simulink model "AFDNFSmodelSPA"  (R2017b)
settings: Solver=ode45  StartTime=0.0  StopTime=1400  FixedStep=1e-3  RelTol=1e-8  EnableMultiTasking=on
PostLoadFcn:
  | run('Methods/NFSOnLoad');
InitFcn:
  | run('Methods/AFDSimInit')
StopFcn:
  | run('Methods/NFSOnLoad');
values from neighbouring files (symbols this model uses):
  nfs = TransferFunction('Plot','true')    [Main.m]    (also in NFSDatabase.sldd = SI
                Imperial
                28184.4409185639)
undefined symbols (not defined in the file or in its folder): Continuous, desired, Earth, F, K_lat, K_long, Kobsvlat, Kobsvlong, lat, latsys, Light, long, longsys, MIL, Newton, Raphson, sigbuilder_block, Time, WGS84
libraries: simulink x6, aerolibtransform2 x2, aerolibwind2 x2, ModelsLibrary x1, ctrlSharedLib x1, sharedutil x1
(part 4 of 4)

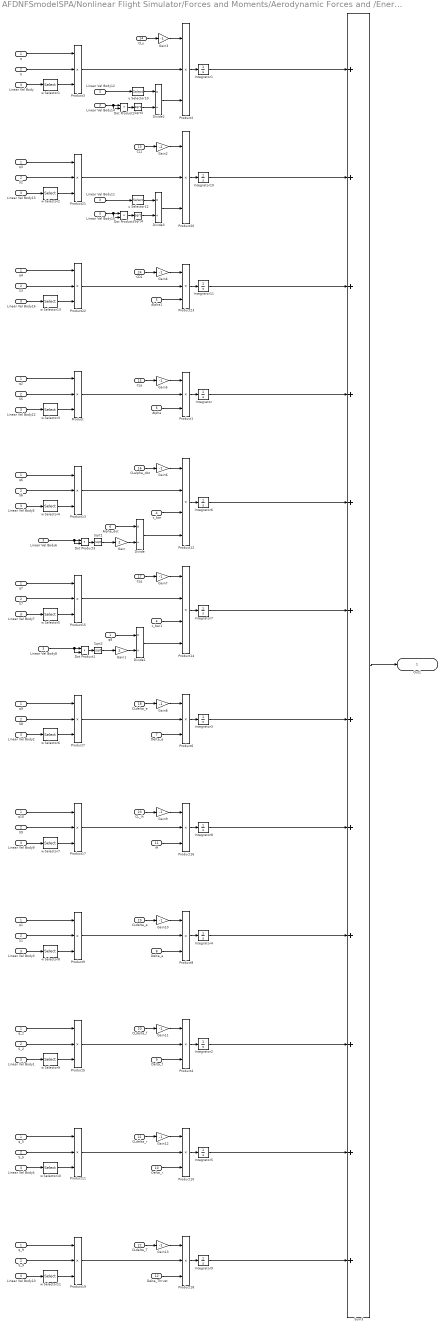
== system AFDNFSmodelSPA/Nonlinear Flight Simulator/Forces and Moments/Aerodynamic Forces and /Energy Analysis1/Longitudinal1/Lift ==
  q : Inport
  S : Inport  Port=2
  Linear Vel Body : Inport  Port=3
  c_bar : Inport  Port=4
  Alpha : Inport  Port=5
  Alpha_dot : Inport  Port=6
  Delta_e : Inport  Port=7
  Delta_a : Inport  Port=8
  Delta_f : Inport  Port=9
  Delta_r : Inport  Port=10
  iH : Inport  Port=11
  Delta_Thrust : Inport  Port=12
  CL1 : Inport  Port=13
  CLu : Inport  Port=14
  CLa : Inport  Port=15
  CLalpha_dot : Inport  Port=16
  CLq : Inport  Port=17
  CLdelta_e : Inport  Port=18
  CLdelta_a : Inport  Port=19
  CLdelta_f : Inport  Port=20
  CLdelta_r : Inport  Port=21
  CLdelta_T : Inport  Port=22
  CL_ih : Inport  Port=23
  CD1 : Inport  Port=24
  Alpha1 : InportShadow  Port=5
  Divide{,1..3} (4 alike) : Product  Inputs=*/
  Dot Product{1..4} (4 alike) : DotProduct  InputSameDT=on  OutDataTypeStr=Inherit: Inherit via internal rule
  Gain : Gain  Gain=2
  Gain1 : Gain  Gain=2
  Gain{3..13} (11 alike) : Gain  Gain=-1
  Gain2 : Gain  Gain=-2
  Integrator{,1..11} (12 alike) : Integrator
  Linear Vel Body{1..16,22} (17 alike) : InportShadow  Port=3
  Product{,1..11,13,15..23} (22 alike) : Product  Inputs=3
  Product12 : Product  Inputs=4
  Product14 : Product  Inputs=4
  S{1..3,5..9} (8 alike) : InportShadow  Port=2
  S_2 : InportShadow  Port=2
  S_5 : InportShadow  Port=2
  S_9 : InportShadow  Port=2
  Sqrt{1..4} (4 alike) : Sqrt  SaturateOnIntegerOverflow=on
  Sum3 : Sum  Inputs=++++++++++++
  c_bar1 : InportShadow  Port=4
  q{1..4,6..10} (9 alike) : InportShadow
  q_2 : InportShadow
  q_5 : InportShadow
  q_9 : InportShadow
  u Selector10 : Selector  InputPortWidth=3  IndexOptions=Index vector (dialog)  Indices=[1]  OutputSizes=1
  u Selector12 : Selector  InputPortWidth=3  IndexOptions=Index vector (dialog)  Indices=[1]  OutputSizes=1
  w Selector{1..11,13} (12 alike) : Selector  InputPortWidth=3  IndexOptions=Index vector (dialog)  Indices=[3]  OutputSizes=1
  Out1 : Outport
  wires:
  Integrator1/1 -> Sum3/1
  CLu/1 -> Gain3/1
  Product3/1 -> Product2/2
  Divide2/1 -> Product2/3
  Product2/1 -> Integrator1/1
  Integrator10/1 -> Sum3/2
  q/1 -> Product3/1
  S/1 -> Product3/2
  Sum3/1 -> Out1/1
  w Selector1/1 -> Product3/3
  Linear Vel Body/1 -> w Selector1/1
  Sqrt3/1 -> Divide2/2
  u Selector10/1 -> Divide2/1
  Dot Product2/1 -> Sqrt3/1
  Linear Vel Body14/1 -> Dot Product2/1, Dot Product2/2
  Linear Vel Body12/1 -> u Selector10/1
  CL1/1 -> Gain2/1
  Product21/1 -> Product20/2
  Divide3/1 -> Product20/3
  Product20/1 -> Integrator10/1
  q3/1 -> Product21/1
  S2/1 -> Product21/2
  w Selector2/1 -> Product21/3
  Linear Vel Body13/1 -> w Selector2/1
  Sqrt4/1 -> Divide3/2
  u Selector12/1 -> Divide3/1
  Dot Product4/1 -> Sqrt4/1
  Linear Vel Body15/1 -> Dot Product4/2, Dot Product4/1
  Linear Vel Body11/1 -> u Selector12/1
  Gain2/1 -> Product20/1
  Integrator6/1 -> Sum3/5
  Integrator3/1 -> Sum3/7
  Integrator4/1 -> Sum3/9
  Integrator2/1 -> Sum3/10
  Integrator5/1 -> Sum3/11
  CLdelta_T/1 -> Gain13/1
  Product19/1 -> Product18/2
  Delta_Thrust/1 -> Product18/3
  Product18/1 -> Integrator9/1
  q_9/1 -> Product19/1
  S_9/1 -> Product19/2
  w Selector11/1 -> Product19/3
  Linear Vel Body10/1 -> w Selector11/1
  Integrator9/1 -> Sum3/12
  CLdelta_r/1 -> Gain12/1
  Product11/1 -> Product10/2
  Delta_r/1 -> Product10/3
  Product10/1 -> Integrator5/1
  q_5/1 -> Product11/1
  S_5/1 -> Product11/2
  w Selector10/1 -> Product11/3
  Linear Vel Body4/1 -> w Selector10/1
  CLdelta_f/1 -> Gain11/1
  Product5/1 -> Product4/2
  Delta_f/1 -> Product4/3
  Product4/1 -> Integrator2/1
  q_2/1 -> Product5/1
  S_2/1 -> Product5/2
  w Selector9/1 -> Product5/3
  Linear Vel Body1/1 -> w Selector9/1
  Alpha/1 -> Product1/3
  CLa/1 -> Gain5/1
  Product/1 -> Product1/2
  Product1/1 -> Integrator/1
  q2/1 -> Product/1
  S5/1 -> Product/2
  Linear Vel Body22/1 -> w Selector3/1
  w Selector3/1 -> Product/3
  CLdelta_e/1 -> Gain8/1
  Product7/1 -> Product6/2
  Delta_e/1 -> Product6/3
  Product6/1 -> Integrator3/1
  q9/1 -> Product7/1
  S8/1 -> Product7/2
  w Selector6/1 -> Product7/3
  Linear Vel Body2/1 -> w Selector6/1
  CLdelta_a/1 -> Gain10/1
  Product9/1 -> Product8/2
  Delta_a/1 -> Product8/3
  Product8/1 -> Integrator4/1
  q1/1 -> Product9/1
  S1/1 -> Product9/2
  w Selector8/1 -> Product9/3
  Linear Vel Body3/1 -> w Selector8/1
  CLalpha_dot/1 -> Gain6/1
  Product13/1 -> Product12/2
  c_bar/1 -> Product12/3
  Product12/1 -> Integrator6/1
  q6/1 -> Product13/1
  S6/1 -> Product13/2
  w Selector4/1 -> Product13/3
  Linear Vel Body5/1 -> w Selector4/1
  Gain/1 -> Divide/2
  Alpha_dot/1 -> Divide/1
  Divide/1 -> Product12/4
  Dot Product3/1 -> Sqrt1/1
  Linear Vel Body6/1 -> Dot Product3/1, Dot Product3/2
  Sqrt1/1 -> Gain/1
  CLq/1 -> Gain7/1
  Product15/1 -> Product14/2
  c_bar1/1 -> Product14/3
  Product14/1 -> Integrator7/1
  q7/1 -> Product15/1
  S7/1 -> Product15/2
  w Selector5/1 -> Product15/3
  Linear Vel Body7/1 -> w Selector5/1
  Gain1/1 -> Divide1/2
  q8/1 -> Divide1/1
  Divide1/1 -> Product14/4
  Dot Product1/1 -> Sqrt2/1
  Linear Vel Body8/1 -> Dot Product1/2, Dot Product1/1
  Sqrt2/1 -> Gain1/1
  CL_ih/1 -> Gain9/1
  Product17/1 -> Product16/2
  iH/1 -> Product16/3
  Product16/1 -> Integrator8/1
  q10/1 -> Product17/1
  S9/1 -> Product17/2
  w Selector7/1 -> Product17/3
  Linear Vel Body9/1 -> w Selector7/1
  Integrator8/1 -> Sum3/8
  Integrator/1 -> Sum3/4
  Integrator7/1 -> Sum3/6
  Alpha1/1 -> Product23/3
  CD1/1 -> Gain4/1
  Product22/1 -> Product23/2
  Product23/1 -> Integrator11/1
  q4/1 -> Product22/1
  S3/1 -> Product22/2
  Linear Vel Body16/1 -> w Selector13/1
  w Selector13/1 -> Product22/3
  Integrator11/1 -> Sum3/3
  Gain3/1 -> Product2/1
  Gain4/1 -> Product23/1
  Gain5/1 -> Product1/1
  Gain6/1 -> Product12/1
  Gain7/1 -> Product14/1
  Gain8/1 -> Product6/1
  Gain9/1 -> Product16/1
  Gain10/1 -> Product8/1
  Gain11/1 -> Product4/1
  Gain12/1 -> Product10/1
  Gain13/1 -> Product18/1

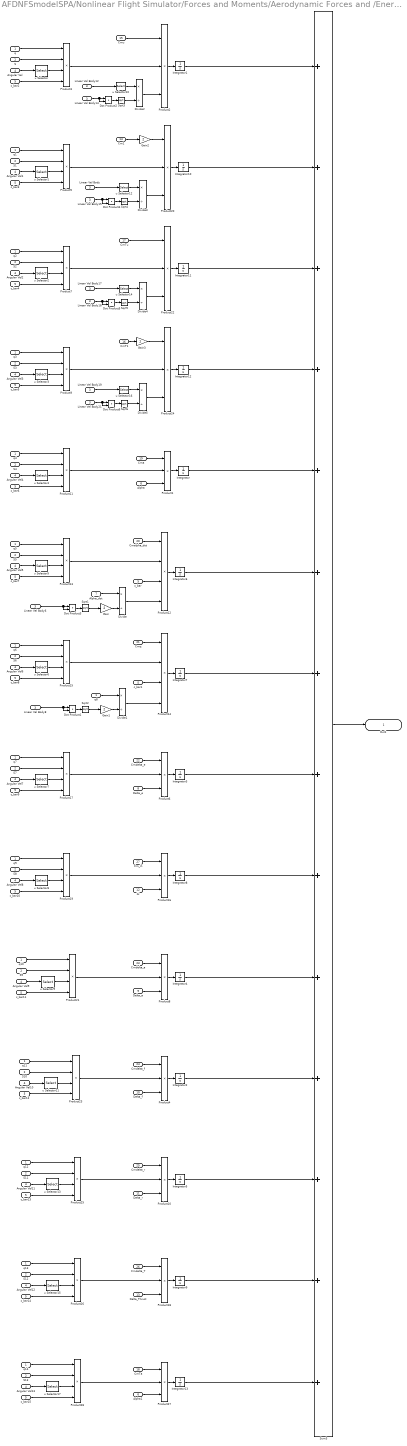
== system AFDNFSmodelSPA/Nonlinear Flight Simulator/Forces and Moments/Aerodynamic Forces and /Energy Analysis1/Longitudinal1/Pitch ==
  q : Inport
  S : Inport  Port=2
  Linear Vel Body : Inport  Port=3
  Angular Vel : Inport  Port=4
  c_bar : Inport  Port=5
  Alpha : Inport  Port=6
  Alpha_dot : Inport  Port=7
  Delta_e : Inport  Port=8
  Delta_a : Inport  Port=9
  Delta_f : Inport  Port=10
  Delta_r : Inport  Port=11
  iH : Inport  Port=12
  Delta_Thrust : Inport  Port=13
  Cm1 : Inport  Port=14
  Cmu : Inport  Port=15
  CmT1 : Inport  Port=16
  CmTu : Inport  Port=17
  CmTa : Inport  Port=18
  Cma : Inport  Port=19
  Cmalpha_dot : Inport  Port=20
  Cmq : Inport  Port=21
  Cmdelta_e : Inport  Port=22
  Cmdelta_a : Inport  Port=23
  Cmdelta_f : Inport  Port=24
  Cmdelta_r : Inport  Port=25
  Cmdelta_T : Inport  Port=26
  Cm_ih : Inport  Port=27
  Alpha1 : InportShadow  Port=6
  Angular Vel{1..13} (13 alike) : InportShadow  Port=4
  Divide{,1..5} (6 alike) : Product  Inputs=*/
  Dot Product{1..6} (6 alike) : DotProduct  InputSameDT=on  OutDataTypeStr=Inherit: Inherit via internal rule
  Gain{,1..3} (4 alike) : Gain  Gain=2
  Integrator{,1..13} (14 alike) : Integrator
  Linear Vel Body{6,8,12,14..15,17..19,21} (9 alike) : InportShadow  Port=3
  Product{1..2,4,6,8,10,16,18,20,22,24,27} (12 alike) : Product  Inputs=3
  Product{3,5,7,9,11..15,17,19,21,23,25..26,28} (16 alike) : Product  Inputs=4
  S{1..13} (13 alike) : InportShadow  Port=2
  Sqrt{1..6} (6 alike) : Sqrt  SaturateOnIntegerOverflow=on
  Sum3 : Sum  Inputs=++++++++++++++
  c_bar{1..15} (15 alike) : InportShadow  Port=5
  q{1..14} (14 alike) : InportShadow
  u Selector{,1..9,11,13,15,17} (14 alike) : Selector  InputPortWidth=3  IndexOptions=Index vector (dialog)  Indices=[2]  OutputSizes=1
  u Selector{10,12,14,16} (4 alike) : Selector  InputPortWidth=3  IndexOptions=Index vector (dialog)  Indices=[1]  OutputSizes=1
  Out1 : Outport
  wires:
  Integrator7/1 -> Sum3/7
  Integrator12/1 -> Sum3/4
  Gain3/1 -> Product24/1
  Linear Vel Body19/1 -> u Selector16/1
  Linear Vel Body21/1 -> Dot Product6/1, Dot Product6/2
  Dot Product6/1 -> Sqrt6/1
  u Selector16/1 -> Divide5/1
  Sqrt6/1 -> Divide5/2
  Product24/1 -> Integrator12/1
  Divide5/1 -> Product24/3
  Product9/1 -> Product24/2
  CmT1/1 -> Gain3/1
  Integrator11/1 -> Sum3/3
  Linear Vel Body17/1 -> u Selector14/1
  Linear Vel Body18/1 -> Dot Product5/2, Dot Product5/1
  Dot Product5/1 -> Sqrt5/1
  u Selector14/1 -> Divide4/1
  Sqrt5/1 -> Divide4/2
  Product22/1 -> Integrator11/1
  Divide4/1 -> Product22/3
  Product7/1 -> Product22/2
  CmTu/1 -> Product22/1
  Gain2/1 -> Product20/1
  Linear Vel Body/1 -> u Selector12/1
  Linear Vel Body15/1 -> Dot Product4/1, Dot Product4/2
  Dot Product4/1 -> Sqrt4/1
  u Selector12/1 -> Divide3/1
  Sqrt4/1 -> Divide3/2
  Product20/1 -> Integrator10/1
  Divide3/1 -> Product20/3
  Product5/1 -> Product20/2
  Cm1/1 -> Gain2/1
  Integrator/1 -> Sum3/5
  Integrator8/1 -> Sum3/9
  Product16/1 -> Integrator8/1
  iH/1 -> Product16/3
  Product19/1 -> Product16/2
  Cm_ih/1 -> Product16/1
  Sqrt2/1 -> Gain1/1
  Linear Vel Body8/1 -> Dot Product1/1, Dot Product1/2
  Dot Product1/1 -> Sqrt2/1
  Divide1/1 -> Product14/4
  q8/1 -> Divide1/1
  Gain1/1 -> Divide1/2
  Product14/1 -> Integrator7/1
  c_bar1/1 -> Product14/3
  Product15/1 -> Product14/2
  Cmq/1 -> Product14/1
  Sqrt1/1 -> Gain/1
  Linear Vel Body6/1 -> Dot Product3/2, Dot Product3/1
  Dot Product3/1 -> Sqrt1/1
  Divide/1 -> Product12/4
  Alpha_dot/1 -> Divide/1
  Gain/1 -> Divide/2
  Product12/1 -> Integrator6/1
  c_bar/1 -> Product12/3
  Product13/1 -> Product12/2
  Cmalpha_dot/1 -> Product12/1
  Product8/1 -> Integrator4/1
  Delta_a/1 -> Product8/3
  Product21/1 -> Product8/2
  Cmdelta_a/1 -> Product8/1
  Product6/1 -> Integrator3/1
  Delta_e/1 -> Product6/3
  Product17/1 -> Product6/2
  Cmdelta_e/1 -> Product6/1
  Product1/1 -> Integrator/1
  Product11/1 -> Product1/2
  Cma/1 -> Product1/1
  Alpha/1 -> Product1/3
  Product4/1 -> Integrator2/1
  Delta_f/1 -> Product4/3
  Product23/1 -> Product4/2
  Cmdelta_f/1 -> Product4/1
  Product10/1 -> Integrator5/1
  Delta_r/1 -> Product10/3
  Product25/1 -> Product10/2
  Cmdelta_r/1 -> Product10/1
  Integrator9/1 -> Sum3/13
  Product18/1 -> Integrator9/1
  Delta_Thrust/1 -> Product18/3
  Product26/1 -> Product18/2
  Cmdelta_T/1 -> Product18/1
  Integrator5/1 -> Sum3/12
  Integrator2/1 -> Sum3/11
  Integrator4/1 -> Sum3/10
  Integrator3/1 -> Sum3/8
  Integrator6/1 -> Sum3/6
  Linear Vel Body12/1 -> u Selector10/1
  Linear Vel Body14/1 -> Dot Product2/2, Dot Product2/1
  Dot Product2/1 -> Sqrt3/1
  u Selector10/1 -> Divide2/1
  Sqrt3/1 -> Divide2/2
  Angular Vel/1 -> u Selector/1
  u Selector/1 -> Product3/3
  Sum3/1 -> Out1/1
  S/1 -> Product3/2
  q/1 -> Product3/1
  Integrator10/1 -> Sum3/2
  Product2/1 -> Integrator1/1
  Divide2/1 -> Product2/3
  Product3/1 -> Product2/2
  Integrator1/1 -> Sum3/1
  CmTa/1 -> Product27/1
  Product28/1 -> Product27/2
  Product27/1 -> Integrator13/1
  Alpha1/1 -> Product27/3
  Integrator13/1 -> Sum3/14
  c_bar2/1 -> Product3/4
  Angular Vel1/1 -> u Selector1/1
  u Selector1/1 -> Product5/3
  S1/1 -> Product5/2
  q1/1 -> Product5/1
  c_bar3/1 -> Product5/4
  Angular Vel2/1 -> u Selector2/1
  u Selector2/1 -> Product7/3
  S2/1 -> Product7/2
  q2/1 -> Product7/1
  c_bar4/1 -> Product7/4
  Angular Vel3/1 -> u Selector3/1
  u Selector3/1 -> Product9/3
  S3/1 -> Product9/2
  q3/1 -> Product9/1
  c_bar5/1 -> Product9/4
  Angular Vel4/1 -> u Selector4/1
  u Selector4/1 -> Product11/3
  S4/1 -> Product11/2
  q4/1 -> Product11/1
  c_bar6/1 -> Product11/4
  Angular Vel5/1 -> u Selector5/1
  u Selector5/1 -> Product13/3
  S5/1 -> Product13/2
  q5/1 -> Product13/1
  c_bar7/1 -> Product13/4
  Angular Vel6/1 -> u Selector6/1
  u Selector6/1 -> Product15/3
  S6/1 -> Product15/2
  q6/1 -> Product15/1
  c_bar8/1 -> Product15/4
  Angular Vel7/1 -> u Selector7/1
  u Selector7/1 -> Product17/3
  S7/1 -> Product17/2
  q7/1 -> Product17/1
  c_bar9/1 -> Product17/4
  Angular Vel8/1 -> u Selector8/1
  u Selector8/1 -> Product19/3
  S8/1 -> Product19/2
  q9/1 -> Product19/1
  c_bar10/1 -> Product19/4
  Angular Vel9/1 -> u Selector9/1
  u Selector9/1 -> Product21/3
  S9/1 -> Product21/2
  q10/1 -> Product21/1
  c_bar11/1 -> Product21/4
  Angular Vel10/1 -> u Selector11/1
  u Selector11/1 -> Product23/3
  S10/1 -> Product23/2
  q11/1 -> Product23/1
  c_bar12/1 -> Product23/4
  Angular Vel11/1 -> u Selector13/1
  u Selector13/1 -> Product25/3
  S11/1 -> Product25/2
  q12/1 -> Product25/1
  c_bar13/1 -> Product25/4
  Angular Vel12/1 -> u Selector15/1
  u Selector15/1 -> Product26/3
  S12/1 -> Product26/2
  q13/1 -> Product26/1
  c_bar14/1 -> Product26/4
  Angular Vel13/1 -> u Selector17/1
  u Selector17/1 -> Product28/3
  S13/1 -> Product28/2
  q14/1 -> Product28/1
  c_bar15/1 -> Product28/4
  Cmu/1 -> Product2/1

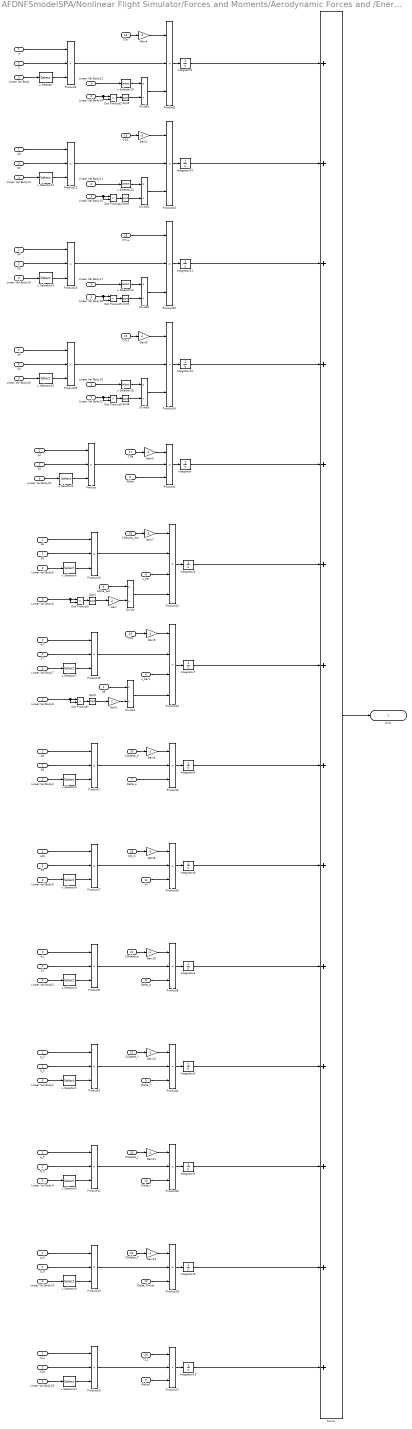
== system AFDNFSmodelSPA/Nonlinear Flight Simulator/Forces and Moments/Aerodynamic Forces and /Energy Analysis1/Longitudinal1/drag ==
  q : Inport
  S : Inport  Port=2
  Linear Vel Body : Inport  Port=3
  c_bar : Inport  Port=4
  Alpha : Inport  Port=5
  Alpha_dot : Inport  Port=6
  Delta_e : Inport  Port=7
  Delta_a : Inport  Port=8
  Delta_f : Inport  Port=9
  Delta_r : Inport  Port=10
  iH : Inport  Port=11
  Delta_Thrust : Inport  Port=12
  CD1 : Inport  Port=13
  CDu : Inport  Port=14
  CTx1 : Inport  Port=15
  CTxu : Inport  Port=16
  CDa : Inport  Port=17
  CDalpha_dot : Inport  Port=18
  CDq : Inport  Port=19
  CDdelta_e : Inport  Port=20
  CDdelta_a : Inport  Port=21
  CDdelta_f : Inport  Port=22
  CDdelta_r : Inport  Port=23
  CDdelta_T : Inport  Port=24
  CD_ih : Inport  Port=25
  CL1 : Inport  Port=26
  Alpha1 : InportShadow  Port=5
  Divide{,1..5} (6 alike) : Product  Inputs=*/
  Dot Product{1..6} (6 alike) : DotProduct  InputSameDT=on  OutDataTypeStr=Inherit: Inherit via internal rule
  Gain : Gain  Gain=2
  Gain1 : Gain  Gain=2
  Gain{4..13} (10 alike) : Gain  Gain=-1
  Gain2 : Gain  Gain=-2
  Gain3 : Gain  Gain=2
  Integrator{,1..13} (14 alike) : Integrator
  Linear Vel Body{1..23} (23 alike) : InportShadow  Port=3
  Product{,1..11,13,15..27} (26 alike) : Product  Inputs=3
  Product12 : Product  Inputs=4
  Product14 : Product  Inputs=4
  S{1..10} (10 alike) : InportShadow  Port=2
  S_2 : InportShadow  Port=2
  S_5 : InportShadow  Port=2
  S_9 : InportShadow  Port=2
  Sqrt{1..6} (6 alike) : Sqrt  SaturateOnIntegerOverflow=on
  Sum3 : Sum  Inputs=++++++++++++++
  c_bar1 : InportShadow  Port=4
  q{1..11} (11 alike) : InportShadow
  q_2 : InportShadow
  q_5 : InportShadow
  q_9 : InportShadow
  u Selector{,1..17} (18 alike) : Selector  InputPortWidth=3  IndexOptions=Index vector (dialog)  Indices=[1]  OutputSizes=1
  Out1 : Outport
  wires:
  Integrator1/1 -> Sum3/1
  CDu/1 -> Gain4/1
  Product3/1 -> Product2/2
  Divide2/1 -> Product2/3
  Product2/1 -> Integrator1/1
  Integrator10/1 -> Sum3/2
  q/1 -> Product3/1
  S/1 -> Product3/2
  Sum3/1 -> Out1/1
  u Selector/1 -> Product3/3
  Linear Vel Body/1 -> u Selector/1
  Sqrt3/1 -> Divide2/2
  u Selector10/1 -> Divide2/1
  Dot Product2/1 -> Sqrt3/1
  Linear Vel Body14/1 -> Dot Product2/1, Dot Product2/2
  Linear Vel Body12/1 -> u Selector10/1
  Integrator6/1 -> Sum3/6
  Integrator3/1 -> Sum3/8
  Integrator4/1 -> Sum3/10
  Integrator2/1 -> Sum3/11
  Integrator5/1 -> Sum3/12
  CDdelta_T/1 -> Gain13/1
  Product19/1 -> Product18/2
  Delta_Thrust/1 -> Product18/3
  Product18/1 -> Integrator9/1
  q_9/1 -> Product19/1
  S_9/1 -> Product19/2
  u Selector9/1 -> Product19/3
  Linear Vel Body10/1 -> u Selector9/1
  Integrator9/1 -> Sum3/13
  CDdelta_r/1 -> Gain11/1
  Product11/1 -> Product10/2
  Delta_r/1 -> Product10/3
  Product10/1 -> Integrator5/1
  q_5/1 -> Product11/1
  S_5/1 -> Product11/2
  u Selector5/1 -> Product11/3
  Linear Vel Body4/1 -> u Selector5/1
  CDdelta_f/1 -> Gain12/1
  Product5/1 -> Product4/2
  Delta_f/1 -> Product4/3
  Product4/1 -> Integrator2/1
  q_2/1 -> Product5/1
  S_2/1 -> Product5/2
  u Selector1/1 -> Product5/3
  Linear Vel Body1/1 -> u Selector1/1
  Alpha/1 -> Product1/3
  CDa/1 -> Gain5/1
  Product/1 -> Product1/2
  Product1/1 -> Integrator/1
  q2/1 -> Product/1
  S5/1 -> Product/2
  Linear Vel Body22/1 -> u Selector2/1
  u Selector2/1 -> Product/3
  CDdelta_e/1 -> Gain6/1
  Product7/1 -> Product6/2
  Delta_e/1 -> Product6/3
  Product6/1 -> Integrator3/1
  q9/1 -> Product7/1
  S8/1 -> Product7/2
  u Selector3/1 -> Product7/3
  Linear Vel Body2/1 -> u Selector3/1
  CDdelta_a/1 -> Gain10/1
  Product9/1 -> Product8/2
  Delta_a/1 -> Product8/3
  Product8/1 -> Integrator4/1
  q1/1 -> Product9/1
  S1/1 -> Product9/2
  u Selector4/1 -> Product9/3
  Linear Vel Body3/1 -> u Selector4/1
  CDalpha_dot/1 -> Gain7/1
  Product13/1 -> Product12/2
  c_bar/1 -> Product12/3
  Product12/1 -> Integrator6/1
  q6/1 -> Product13/1
  S6/1 -> Product13/2
  u Selector6/1 -> Product13/3
  Linear Vel Body5/1 -> u Selector6/1
  Gain/1 -> Divide/2
  Alpha_dot/1 -> Divide/1
  Divide/1 -> Product12/4
  Dot Product3/1 -> Sqrt1/1
  Linear Vel Body6/1 -> Dot Product3/1, Dot Product3/2
  Sqrt1/1 -> Gain/1
  CDq/1 -> Gain9/1
  Product15/1 -> Product14/2
  c_bar1/1 -> Product14/3
  Product14/1 -> Integrator7/1
  q7/1 -> Product15/1
  S7/1 -> Product15/2
  u Selector7/1 -> Product15/3
  Linear Vel Body7/1 -> u Selector7/1
  Gain1/1 -> Divide1/2
  q8/1 -> Divide1/1
  Divide1/1 -> Product14/4
  Dot Product1/1 -> Sqrt2/1
  Linear Vel Body8/1 -> Dot Product1/2, Dot Product1/1
  Sqrt2/1 -> Gain1/1
  CD_ih/1 -> Gain8/1
  Product17/1 -> Product16/2
  iH/1 -> Product16/3
  Product16/1 -> Integrator8/1
  q10/1 -> Product17/1
  S9/1 -> Product17/2
  u Selector8/1 -> Product17/3
  Linear Vel Body9/1 -> u Selector8/1
  Integrator8/1 -> Sum3/9
  Integrator/1 -> Sum3/5
  CD1/1 -> Gain2/1
  Product21/1 -> Product20/2
  Divide3/1 -> Product20/3
  Product20/1 -> Integrator10/1
  q3/1 -> Product21/1
  S2/1 -> Product21/2
  u Selector11/1 -> Product21/3
  Linear Vel Body13/1 -> u Selector11/1
  Sqrt4/1 -> Divide3/2
  u Selector12/1 -> Divide3/1
  Dot Product4/1 -> Sqrt4/1
  Linear Vel Body15/1 -> Dot Product4/2, Dot Product4/1
  Linear Vel Body11/1 -> u Selector12/1
  Gain2/1 -> Product20/1
  CTxu/1 -> Product22/1
  Product23/1 -> Product22/2
  Divide4/1 -> Product22/3
  Product22/1 -> Integrator11/1
  q4/1 -> Product23/1
  S3/1 -> Product23/2
  u Selector13/1 -> Product23/3
  Linear Vel Body16/1 -> u Selector13/1
  Sqrt5/1 -> Divide4/2
  u Selector14/1 -> Divide4/1
  Dot Product5/1 -> Sqrt5/1
  Linear Vel Body18/1 -> Dot Product5/1, Dot Product5/2
  Linear Vel Body17/1 -> u Selector14/1
  Integrator11/1 -> Sum3/3
  CTx1/1 -> Gain3/1
  Product25/1 -> Product24/2
  Divide5/1 -> Product24/3
  Product24/1 -> Integrator12/1
  q5/1 -> Product25/1
  S4/1 -> Product25/2
  u Selector15/1 -> Product25/3
  Linear Vel Body20/1 -> u Selector15/1
  Sqrt6/1 -> Divide5/2
  u Selector16/1 -> Divide5/1
  Dot Product6/1 -> Sqrt6/1
  Linear Vel Body21/1 -> Dot Product6/2, Dot Product6/1
  Linear Vel Body19/1 -> u Selector16/1
  Gain3/1 -> Product24/1
  Integrator12/1 -> Sum3/4
  Integrator7/1 -> Sum3/7
  Alpha1/1 -> Product27/3
  CL1/1 -> Product27/1
  Product26/1 -> Product27/2
  Product27/1 -> Integrator13/1
  q11/1 -> Product26/1
  S10/1 -> Product26/2
  Linear Vel Body23/1 -> u Selector17/1
  u Selector17/1 -> Product26/3
  Integrator13/1 -> Sum3/14
  Gain4/1 -> Product2/1
  Gain5/1 -> Product1/1
  Gain6/1 -> Product6/1
  Gain7/1 -> Product12/1
  Gain9/1 -> Product14/1
  Gain8/1 -> Product16/1
  Gain10/1 -> Product8/1
  Gain12/1 -> Product4/1
  Gain11/1 -> Product10/1
  Gain13/1 -> Product18/1

== system AFDNFSmodelSPA/Nonlinear Flight Simulator/Forces and Moments/Aerodynamic Forces and /Forces/Aerodynamic Forces/Wind2Body TM ==
  Alpha : Inport  PortDimensions=1
  Beta : Inport  Port=2  PortDimensions=1
  ChSign : Gain  Gain=-1  SaturateOnIntegerOverflow=on  OutDataTypeStr=Inherit: Same as input  ParamDataTypeStr=Inherit: Same as input
  ChSign1 : Gain  Gain=-1  SaturateOnIntegerOverflow=on  OutDataTypeStr=Inherit: Same as input  ParamDataTypeStr=Inherit: Same as input
  ChSign2 : Gain  Gain=-1  SaturateOnIntegerOverflow=on  OutDataTypeStr=Inherit: Same as input  ParamDataTypeStr=Inherit: Same as input
  Product{,1..3} (4 alike) : Product  SaturateOnIntegerOverflow=on  InputSameDT=on  OutDataTypeStr=Inherit: Same as first input
  S Matrix : Concatenate  NumInputs=3  Mode=Multidimensional array  ConcatenateDimension=2
  S Col1 : Concatenate  NumInputs=3  Mode=Multidimensional array
  S Col2 : Concatenate  NumInputs=3  Mode=Multidimensional array
  S Col3 : Concatenate  NumInputs=3  Mode=Multidimensional array
  Trigonometric Function : Trigonometry
  Trigonometric Function1 : Trigonometry  Operator=cos
  Trigonometric Function2 : Trigonometry
  Trigonometric Function3 : Trigonometry  Operator=cos
  Zero : Constant  Value=0
  T_BW : Outport  PortDimensions=[3,3]
  wires:
  S Matrix/1 -> T_BW/1
  S Col3/1 -> S Matrix/3
  S Col2/1 -> S Matrix/2
  S Col1/1 -> S Matrix/1
  ChSign2/1 -> S Col3/2
  Product2/1 -> S Col3/1
  Product3/1 -> ChSign2/1
  Zero/1 -> S Col2/3
  ChSign1/1 -> S Col1/3
  ChSign/1 -> S Col1/2
  Product/1 -> S Col1/1
  Product1/1 -> ChSign/1
  Trigonometric Function3/1 -> Product2/2, S Col2/2, Product/2
  Trigonometric Function2/1 -> Product3/2, S Col2/1, Product1/2
  Trigonometric Function1/1 -> Product/1, S Col3/3, Product1/1
  Trigonometric Function/1 -> Product3/1, Product2/1, ChSign1/1
  Beta/1 -> Trigonometric Function2/1, Trigonometric Function3/1
  Alpha/1 -> Trigonometric Function1/1, Trigonometric Function/1

== system AFDNFSmodelSPA/Nonlinear Flight Simulator/Forces and Moments/Aerodynamic Forces and /Forces/Force Coefficients Calculator/Drag Coefficient ==
  CL : Inport  PortDimensions=1
  alpha : Inport  Port=2  PortDimensions=1
  DeltaElevator : Inport  Port=3  PortDimensions=1
  DeltaFlap : Inport  Port=4  PortDimensions=1
  DeltaAileron : Inport  Port=5  PortDimensions=1
  DeltaRudder : Inport  Port=6  PortDimensions=1
  Mach : Inport  Port=7  PortDimensions=1
  Abs{,1..4} (5 alike) : Abs  SaturateOnIntegerOverflow=on
  CD0 : Constant  Value=cD0
  CL^2 : Math  Operator=square  SaturateOnIntegerOverflow=on
  Induced Drag : Gain  Gain=nfs.aero.k  SaturateOnIntegerOverflow=on  OutDataTypeStr=Inherit: Same as input  ParamDataTypeStr=Inherit: Same as input
  Sum2 : Sum  Inputs=++++++++  SaturateOnIntegerOverflow=on  InputSameDT=on  OutDataTypeStr=Inherit: Same as first input
  cDM : Gain  Gain=nfs.aero.cDM  SaturateOnIntegerOverflow=on  OutDataTypeStr=Inherit: Same as input  ParamDataTypeStr=Inherit: Same as input
  cDalpha : Gain  Gain=nfs.aero.cDalpha  SaturateOnIntegerOverflow=on  OutDataTypeStr=Inherit: Same as input  ParamDataTypeStr=Inherit: Same as input
  cDdelta_a : Gain  Gain=nfs.aero.cDdelta_a  SaturateOnIntegerOverflow=on  OutDataTypeStr=Inherit: Same as input  ParamDataTypeStr=Inherit: Same as input
  cDdelta_e : Gain  Gain=nfs.aero.cDdelta_e  SaturateOnIntegerOverflow=on  OutDataTypeStr=Inherit: Same as input  ParamDataTypeStr=Inherit: Same as input
  cDdelta_f : Gain  Gain=nfs.aero.cDdelta_f  SaturateOnIntegerOverflow=on  OutDataTypeStr=Inherit: Same as input  ParamDataTypeStr=Inherit: Same as input
  cDdelta_r : Gain  Gain=nfs.aero.cDdelta_r  SaturateOnIntegerOverflow=on  OutDataTypeStr=Inherit: Same as input  ParamDataTypeStr=Inherit: Same as input
  CD : Outport  PortDimensions=1
  wires:
  Sum2/1 -> CD/1
  DeltaRudder/1 -> cDdelta_r/1
  DeltaAileron/1 -> cDdelta_a/1
  DeltaElevator/1 -> cDdelta_e/1
  DeltaFlap/1 -> cDdelta_f/1
  Mach/1 -> cDM/1
  CL/1 -> CL^2/1
  cDdelta_r/1 -> Abs3/1
  cDdelta_a/1 -> Abs2/1
  cDdelta_e/1 -> Abs1/1
  cDdelta_f/1 -> Abs/1
  Induced Drag/1 -> Sum2/2
  CD0/1 -> Sum2/1
  CL^2/1 -> Induced Drag/1
  alpha/1 -> cDalpha/1
  cDalpha/1 -> Abs4/1
  Abs/1 -> Sum2/4
  Abs1/1 -> Sum2/5
  Abs2/1 -> Sum2/6
  Abs3/1 -> Sum2/7
  cDM/1 -> Sum2/8
  Abs4/1 -> Sum2/3

== system AFDNFSmodelSPA/Nonlinear Flight Simulator/Forces and Moments/Aerodynamic Forces and /Forces/Force Coefficients Calculator/Lift Coefficient ==
  Linear Velocity : Inport  PortDimensions=[3 1]
  Alpha : Inport  Port=2  PortDimensions=1
  DeltaElevator : Inport  Port=3  PortDimensions=1
  DeltaFlap : Inport  Port=4  PortDimensions=1
  Alphadot : Inport  Port=5  PortDimensions=1
  Q : Inport  Port=6  PortDimensions=1
  Mach : Inport  Port=7  PortDimensions=1
  1 : Gain  Gain=2  SaturateOnIntegerOverflow=on  OutDataTypeStr=Inherit: Same as input  ParamDataTypeStr=Inherit: Same as input
  CL*c/(2V) : Product  Inputs=**/  SaturateOnIntegerOverflow=on  InputSameDT=on  OutDataTypeStr=Inherit: Same as first input
  CL0 : Constant  Value=cL0
  CLM : Gain  Gain=nfs.aero.cLM  SaturateOnIntegerOverflow=on  OutDataTypeStr=Inherit: Same as input  ParamDataTypeStr=Inherit: Same as input
  Sum1 : Sum  SaturateOnIntegerOverflow=on  InputSameDT=on  OutDataTypeStr=Inherit: Same as first input
  Sum3 : Sum  Inputs=++++++  SaturateOnIntegerOverflow=on  InputSameDT=on  OutDataTypeStr=Inherit: Same as first input
  Velocity Magnitude : Subsystem
  Wing chord1 : Constant  Value=meanchord
  cLalpha : Gain  Gain=nfs.aero.cLalpha  SaturateOnIntegerOverflow=on  OutDataTypeStr=Inherit: Same as input  ParamDataTypeStr=Inherit: Same as input
  cLalphadot : Gain  Gain=nfs.aero.cLalphadot  SaturateOnIntegerOverflow=on  OutDataTypeStr=Inherit: Same as input  ParamDataTypeStr=Inherit: Same as input
  cLdelta_e : Gain  Gain=nfs.aero.cLdelta_e  SaturateOnIntegerOverflow=on  OutDataTypeStr=Inherit: Same as input  ParamDataTypeStr=Inherit: Same as input
  cLdelta_f : Gain  Gain=nfs.aero.cLdelta_f  SaturateOnIntegerOverflow=on  OutDataTypeStr=Inherit: Same as input  ParamDataTypeStr=Inherit: Same as input
  cLq : Gain  Gain=nfs.aero.cLq  SaturateOnIntegerOverflow=on  OutDataTypeStr=Inherit: Same as input  ParamDataTypeStr=Inherit: Same as input
  CL : Outport  PortDimensions=1
  wires:
  Sum3/1 -> CL/1
  Q/1 -> cLq/1
  Alphadot/1 -> cLalphadot/1
  Velocity Magnitude/1(Velocity Magnitude) -> 1/1
  Linear Velocity/1 -> Velocity Magnitude/1(Velocity)
  Mach/1 -> CLM/1
  CL*c/(2V)/1 -> Sum3/5
  cLdelta_f/1 -> Sum3/4
  cLdelta_e/1 -> Sum3/3
  cLalpha/1 -> Sum3/2
  CL0/1 -> Sum3/1
  Sum1/1 -> CL*c/(2V)/1
  cLalphadot/1 -> Sum1/1
  DeltaFlap/1 -> cLdelta_f/1
  DeltaElevator/1 -> cLdelta_e/1
  Alpha/1 -> cLalpha/1
  cLq/1 -> Sum1/2
  Wing chord1/1 -> CL*c/(2V)/2
  1/1 -> CL*c/(2V)/3
  CLM/1 -> Sum3/6

== system AFDNFSmodelSPA/Nonlinear Flight Simulator/Forces and Moments/Aerodynamic Forces and /Forces/Force Coefficients Calculator/SideForce Coefficient ==
  Linear Velocity : Inport  PortDimensions=[3 1]
  Beta : Inport  Port=2  PortDimensions=1
  P : Inport  Port=3  PortDimensions=1
  R : Inport  Port=4  PortDimensions=1
  DeltaAileron : Inport  Port=5  PortDimensions=1
  DeltaRudder : Inport  Port=6  PortDimensions=1
  2 : Gain  Gain=2  SaturateOnIntegerOverflow=on  OutDataTypeStr=Inherit: Same as input  ParamDataTypeStr=Inherit: Same as input
  CY*b/(2V) : Product  Inputs=**/  SaturateOnIntegerOverflow=on  InputSameDT=on  OutDataTypeStr=Inherit: Same as first input
  Sum : Sum  SaturateOnIntegerOverflow=on  InputSameDT=on  OutDataTypeStr=Inherit: Same as first input
  Sum2 : Sum  Inputs=++++  SaturateOnIntegerOverflow=on  InputSameDT=on  OutDataTypeStr=Inherit: Same as first input
  Velocity Magnitude : Subsystem
  Wing span : Constant  Value=nfs.span
  cYbeta : Gain  Gain=nfs.aero.cYbeta  SaturateOnIntegerOverflow=on  OutDataTypeStr=Inherit: Same as input  ParamDataTypeStr=Inherit: Same as input
  cYdelta_a : Gain  Gain=nfs.aero.cYdelta_a  SaturateOnIntegerOverflow=on  OutDataTypeStr=Inherit: Same as input  ParamDataTypeStr=Inherit: Same as input
  cYdelta_r : Gain  Gain=nfs.aero.cYdelta_r  SaturateOnIntegerOverflow=on  OutDataTypeStr=Inherit: Same as input  ParamDataTypeStr=Inherit: Same as input
  cYp : Gain  Gain=nfs.aero.cYp  SaturateOnIntegerOverflow=on  OutDataTypeStr=Inherit: Same as input  ParamDataTypeStr=Inherit: Same as input
  cYr : Gain  Gain=nfs.aero.cYr  SaturateOnIntegerOverflow=on  OutDataTypeStr=Inherit: Same as input  ParamDataTypeStr=Inherit: Same as input
  CY : Outport
  wires:
  Sum2/1 -> CY/1
  R/1 -> cYr/1
  P/1 -> cYp/1
  DeltaRudder/1 -> cYdelta_r/1
  DeltaAileron/1 -> cYdelta_a/1
  Velocity Magnitude/1(Velocity Magnitude) -> 2/1
  Linear Velocity/1 -> Velocity Magnitude/1(Velocity)
  Beta/1 -> cYbeta/1
  CY*b/(2V)/1 -> Sum2/4
  cYdelta_r/1 -> Sum2/3
  cYdelta_a/1 -> Sum2/2
  cYbeta/1 -> Sum2/1
  2/1 -> CY*b/(2V)/3
  Wing span/1 -> CY*b/(2V)/2
  Sum/1 -> CY*b/(2V)/1
  cYr/1 -> Sum/2
  cYp/1 -> Sum/1

== system AFDNFSmodelSPA/Nonlinear Flight Simulator/Forces and Moments/Aerodynamic Forces and /Moments/Aerodynamic Moment /Wind2Body TM ==
  Alpha : Inport  PortDimensions=1
  Beta : Inport  Port=2  PortDimensions=1
  ChSign : Gain  Gain=-1  SaturateOnIntegerOverflow=on  OutDataTypeStr=Inherit: Same as input  ParamDataTypeStr=Inherit: Same as input
  ChSign1 : Gain  Gain=-1  SaturateOnIntegerOverflow=on  OutDataTypeStr=Inherit: Same as input  ParamDataTypeStr=Inherit: Same as input
  ChSign2 : Gain  Gain=-1  SaturateOnIntegerOverflow=on  OutDataTypeStr=Inherit: Same as input  ParamDataTypeStr=Inherit: Same as input
  Product{,1..3} (4 alike) : Product  SaturateOnIntegerOverflow=on  InputSameDT=on  OutDataTypeStr=Inherit: Same as first input
  S Matrix : Concatenate  NumInputs=3  Mode=Multidimensional array  ConcatenateDimension=2
  S Col1 : Concatenate  NumInputs=3  Mode=Multidimensional array
  S Col2 : Concatenate  NumInputs=3  Mode=Multidimensional array
  S Col3 : Concatenate  NumInputs=3  Mode=Multidimensional array
  Trigonometric Function : Trigonometry
  Trigonometric Function1 : Trigonometry  Operator=cos
  Trigonometric Function2 : Trigonometry
  Trigonometric Function3 : Trigonometry  Operator=cos
  Zero : Constant  Value=0
  T_BW : Outport  PortDimensions=[3,3]
  wires:
  S Matrix/1 -> T_BW/1
  S Col3/1 -> S Matrix/3
  S Col2/1 -> S Matrix/2
  S Col1/1 -> S Matrix/1
  ChSign2/1 -> S Col3/2
  Product2/1 -> S Col3/1
  Product3/1 -> ChSign2/1
  Zero/1 -> S Col2/3
  ChSign1/1 -> S Col1/3
  ChSign/1 -> S Col1/2
  Product/1 -> S Col1/1
  Product1/1 -> ChSign/1
  Trigonometric Function3/1 -> Product2/2, S Col2/2, Product/2
  Trigonometric Function2/1 -> Product3/2, S Col2/1, Product1/2
  Trigonometric Function1/1 -> Product/1, S Col3/3, Product1/1
  Trigonometric Function/1 -> Product3/1, Product2/1, ChSign1/1
  Beta/1 -> Trigonometric Function2/1, Trigonometric Function3/1
  Alpha/1 -> Trigonometric Function1/1, Trigonometric Function/1

== system AFDNFSmodelSPA/Nonlinear Flight Simulator/Forces and Moments/Aerodynamic Forces and /Moments/Pitch Moment Coefficient/Velocity Magnitude ==
  Velocity : Inport
  Dot Product : DotProduct  InputSameDT=on  OutDataTypeStr=Inherit: Inherit via internal rule
  Sqrt : Sqrt  SaturateOnIntegerOverflow=on
  Velocity Magnitude : Outport
  wires:
  Sqrt/1 -> Velocity Magnitude/1  "abs(V)"
  Velocity/1 -> Dot Product/2, Dot Product/1
  Dot Product/1 -> Sqrt/1

== system AFDNFSmodelSPA/Nonlinear Flight Simulator/Forces and Moments/Aerodynamic Forces and /Moments/Roll Moment Coefficient/Velocity Magnitude ==
  Velocity : Inport
  Dot Product : DotProduct  InputSameDT=on  OutDataTypeStr=Inherit: Inherit via internal rule
  Sqrt : Sqrt  SaturateOnIntegerOverflow=on
  Velocity Magnitude : Outport
  wires:
  Sqrt/1 -> Velocity Magnitude/1  "abs(V)"
  Velocity/1 -> Dot Product/2, Dot Product/1
  Dot Product/1 -> Sqrt/1

== system AFDNFSmodelSPA/Nonlinear Flight Simulator/Forces and Moments/Aerodynamic Forces and /Moments/Yaw Moment Coefficient/Velocity Magnitude ==
  Velocity : Inport
  Dot Product : DotProduct  InputSameDT=on  OutDataTypeStr=Inherit: Inherit via internal rule
  Sqrt : Sqrt  SaturateOnIntegerOverflow=on
  Velocity Magnitude : Outport
  wires:
  Sqrt/1 -> Velocity Magnitude/1  "abs(V)"
  Velocity/1 -> Dot Product/2, Dot Product/1
  Dot Product/1 -> Sqrt/1

== system AFDNFSmodelSPA/Nonlinear Flight Simulator/Forces and Moments/Aerodynamic Forces and /Turbulence/Turbulence Model/Dryden Turbulence Model ==
  In : Inport
  Bus Creator2 : BusCreator  Inputs=2
  Bus Selector1 : BusSelector  OutputSignals=Altitude,Linear Velocity,DCM
  Bus Selector2 : BusSelector  OutputSignals=Linear Velocity,Angular Velocity
  Dryden Wind Turbulence Model (Continuous (+q +r)) : aerolibwind2/Dryden Wind Turbulence Model  (Continuous (+q -r))  units=Metric (MKS)  spec=MIL-F-8785C  model=Continuous Dryden (+q +r)  W20=15  Wdeg=0  TurbProb=10^-2 - Light  L_high=nfs.Uncertainty.Turbulence.Dryden.ScaleLength  Wingspan=nfs.span  ts=nfs.Uncertainty.Noise.SampleTime  Seed=nfs.Uncertainty.Turbulence.Dryden.Seed  T_on=on
      settings: SourceProductName=Aerospace Blockset
  Sum1 : Sum  Inputs=++|
  Sum2 : Sum  Inputs=++|
  Velocity Magnitude : Subsystem
  Out : Outport
  wires:
  Dryden Wind Turbulence Model (Continuous (+q +r))/2 -> Sum2/2
  Bus Creator2/1 -> Out/1
  Bus Selector1/1 -> Dryden Wind Turbulence Model (Continuous (+q +r))/1  "<Altitude>"
  Velocity Magnitude/1(Velocity Magnitude) -> Dryden Wind Turbulence Model (Continuous (+q +r))/2
  In/1 -> Bus Selector1/1, Bus Selector2/1
  Bus Selector1/2 -> Velocity Magnitude/1(Velocity)  "<Linear Velocity>"
  Bus Selector1/3 -> Dryden Wind Turbulence Model (Continuous (+q +r))/3  "<DCM>"
  Dryden Wind Turbulence Model (Continuous (+q +r))/1 -> Sum1/2
  Bus Selector2/2 -> Sum2/1  "<Angular Velocity>"
  Bus Selector2/1 -> Sum1/1  "<Linear Velocity>"
  Sum2/1 -> Bus Creator2/2  "Angular Velocity"
  Sum1/1 -> Bus Creator2/1  "Linear Velocity"

== system AFDNFSmodelSPA/Nonlinear Flight Simulator/Forces and Moments/Aerodynamic Forces and /Turbulence/Turbulence Model/No Turbulence ==
  In : Inport
  Bus Creator1 : BusCreator  Inputs=2
  Bus Selector : BusSelector  OutputSignals=Linear Velocity,Angular Velocity
  Out : Outport
  wires:
  In/1 -> Bus Selector/1
  Bus Creator1/1 -> Out/1
  Bus Selector/2 -> Bus Creator1/2  "<Angular Velocity>"
  Bus Selector/1 -> Bus Creator1/1  "<Linear Velocity>"

== system AFDNFSmodelSPA/Nonlinear Flight Simulator/Forces and Moments/Aerodynamic Forces and /Turbulence/Turbulence Model/Von-Karman Turbulence Model ==
  In : Inport
  Bus Creator2 : BusCreator  Inputs=2
  Bus Selector1 : BusSelector  OutputSignals=Altitude,Linear Velocity,DCM
  Bus Selector2 : BusSelector  OutputSignals=Linear Velocity,Angular Velocity
  Sum1 : Sum  Inputs=++|
  Sum2 : Sum  Inputs=++|
  Velocity Magnitude : Subsystem
  Von Karman Wind Turbulence Model (Continuous (+q +r)) : aerolibwind2/Dryden Wind Turbulence Model  (Continuous (+q -r))  units=Metric (MKS)  spec=MIL-F-8785C  model=Continuous Von Karman (+q +r)  W20=15  Wdeg=0  TurbProb=10^-2 - Light  L_high=nfs.Uncertainty.Turbulence.VonKarman.ScaleLength  Wingspan=nfs.span  ts=nfs.Uncertainty.Noise.SampleTime  Seed=nfs.Uncertainty.Turbulence.VonKarman.Seed  T_on=on
      settings: SourceProductName=Aerospace Blockset
  Out : Outport
  wires:
  Sum1/1 -> Bus Creator2/1  "Linear Velocity"
  Sum2/1 -> Bus Creator2/2  "Angular Velocity"
  Bus Selector2/1 -> Sum1/1  "<Linear Velocity>"
  Bus Selector2/2 -> Sum2/1  "<Angular Velocity>"
  Von Karman Wind Turbulence Model (Continuous (+q +r))/1 -> Sum1/2
  Bus Selector1/3 -> Von Karman Wind Turbulence Model (Continuous (+q +r))/3  "<DCM>"
  Bus Selector1/2 -> Velocity Magnitude/1(Velocity)  "<Linear Velocity>"
  In/1 -> Bus Selector2/1, Bus Selector1/1
  Velocity Magnitude/1(Velocity Magnitude) -> Von Karman Wind Turbulence Model (Continuous (+q +r))/2
  Bus Selector1/1 -> Von Karman Wind Turbulence Model (Continuous (+q +r))/1  "<Altitude>"
  Bus Creator2/1 -> Out/1
  Von Karman Wind Turbulence Model (Continuous (+q +r))/2 -> Sum2/2

== system AFDNFSmodelSPA/Navigation & Sensor System/Navigation Model/01-Test Model/Navigation Model - Simple/Euler angles & Direction Cosine Using Quaternions/Rotation Angles to DCM1/Create Transformation Matrix ==
  M11 : Inport  PortDimensions=1
  M12 : Inport  Port=2  PortDimensions=1
  M13 : Inport  Port=3  PortDimensions=1
  M21 : Inport  Port=4  PortDimensions=1
  M22 : Inport  Port=5  PortDimensions=1
  M23 : Inport  Port=6  PortDimensions=1
  M31 : Inport  Port=7  PortDimensions=1
  M32 : Inport  Port=8  PortDimensions=1
  M33 : Inport  Port=9  PortDimensions=1
  Reshape (9) to [3x3] column-major : Reshape  OutputDimensionality=Customize  OutputDimensions=[3,3]
  Vector Concatenate : Concatenate  NumInputs=9
  Matrix : Outport  PortDimensions=[3 3]
  wires:
  M33/1 -> Vector Concatenate/9
  M23/1 -> Vector Concatenate/8
  M13/1 -> Vector Concatenate/7
  M32/1 -> Vector Concatenate/6
  Reshape (9) to [3x3] column-major/1 -> Matrix/1
  M22/1 -> Vector Concatenate/5
  M12/1 -> Vector Concatenate/4
  M31/1 -> Vector Concatenate/3
  M21/1 -> Vector Concatenate/2
  M11/1 -> Vector Concatenate/1
  Vector Concatenate/1 -> Reshape (9) to [3x3] column-major/1

== system AFDNFSmodelSPA/Navigation & Sensor System/Navigation Model/01-Test Model/Navigation Model - Simple/Euler angles & Direction Cosine Using Quaternions/Rotation Angles to DCM1/Quaternion Normalize ==
  q : Inport
  Demux : Demux
  Demux1 : Demux
  Mux : Mux
  Product{,1..3} (4 alike) : Product  Inputs=*/
  Product{4..7} (4 alike) : Product
  Sum : Sum  Inputs=4
  sqrt : Sqrt  AlgorithmType=Newton-Raphson  SaturateOnIntegerOverflow=on
  normal(q) : Outport
  wires:
  Product3/1 -> Mux/4
  Product2/1 -> Mux/3
  Product1/1 -> Mux/2
  Product/1 -> Mux/1
  sqrt/1 -> Product3/2, Product2/2, Product/2, Product1/2
  q/1 -> Demux/1, Demux1/1
  Mux/1 -> normal(q)/1
  Demux/1 -> Product/1
  Demux/2 -> Product1/1
  Demux/3 -> Product2/1
  Demux/4 -> Product3/1
  Sum/1 -> sqrt/1
  Product4/1 -> Sum/1
  Product5/1 -> Sum/2
  Product6/1 -> Sum/3
  Product7/1 -> Sum/4
  Demux1/1 -> Product4/2, Product4/1
  Demux1/2 -> Product5/2, Product5/1
  Demux1/3 -> Product6/2, Product6/1
  Demux1/4 -> Product7/2, Product7/1

== system AFDNFSmodelSPA/Navigation & Sensor System/Navigation Model/01-Test Model/Navigation Model - Simple/Euler angles & Direction Cosine Using Quaternions/Rotation Angles to DCM1/a11 ==
  normal(q) : Inport
  Demux : Demux
  Product{,1..3} (4 alike) : Product  RndMeth=Zero
  Sum : Sum  Inputs=++--
  A11 : Outport
  wires:
  Sum/1 -> A11/1
  Demux/4 -> Product/2, Product/1
  Demux/3 -> Product1/2, Product1/1
  Demux/2 -> Product2/2, Product2/1
  Demux/1 -> Product3/2, Product3/1
  Product3/1 -> Sum/1
  Product2/1 -> Sum/2
  Product1/1 -> Sum/3
  Product/1 -> Sum/4
  normal(q)/1 -> Demux/1

== system AFDNFSmodelSPA/Navigation & Sensor System/Navigation Model/01-Test Model/Navigation Model - Simple/Euler angles & Direction Cosine Using Quaternions/Rotation Angles to DCM1/a12 ==
  normal(q) : Inport
  Demux : Demux
  Gain : Gain  Gain=2
  Product2 : Product  RndMeth=Zero
  Product3 : Product  RndMeth=Zero
  Sum : Sum  Inputs=|++
  A12 : Outport
  wires:
  Product2/1 -> Sum/2
  Product3/1 -> Sum/1
  Sum/1 -> Gain/1
  Demux/1 -> Product3/2
  Demux/2 -> Product2/1
  Demux/4 -> Product3/1
  Demux/3 -> Product2/2
  normal(q)/1 -> Demux/1
  Gain/1 -> A12/1

== system AFDNFSmodelSPA/Navigation & Sensor System/Navigation Model/01-Test Model/Navigation Model - Simple/Euler angles & Direction Cosine Using Quaternions/Rotation Angles to DCM1/a13 ==
  normal(q) : Inport
  Demux : Demux
  Gain : Gain  Gain=2
  Product1 : Product  RndMeth=Zero
  Product2 : Product  RndMeth=Zero
  Sum : Sum  Inputs=|-+
  A13 : Outport
  wires:
  Demux/1 -> Product1/1
  Product1/1 -> Sum/1
  Product2/1 -> Sum/2
  Demux/4 -> Product2/2
  Demux/2 -> Product2/1
  Demux/3 -> Product1/2
  normal(q)/1 -> Demux/1
  Gain/1 -> A13/1
  Sum/1 -> Gain/1

== system AFDNFSmodelSPA/Navigation & Sensor System/Navigation Model/01-Test Model/Navigation Model - Simple/Euler angles & Direction Cosine Using Quaternions/Rotation Angles to DCM1/a21 ==
  normal(q) : Inport
  Demux : Demux
  Gain : Gain  Gain=2
  Product2 : Product  RndMeth=Zero
  Product3 : Product  RndMeth=Zero
  Sum : Sum  Inputs=|-+
  A21 : Outport
  wires:
  Gain/1 -> A21/1
  normal(q)/1 -> Demux/1
  Demux/3 -> Product2/2
  Demux/4 -> Product3/1
  Demux/2 -> Product2/1
  Demux/1 -> Product3/2
  Sum/1 -> Gain/1
  Product3/1 -> Sum/1
  Product2/1 -> Sum/2

== system AFDNFSmodelSPA/Navigation & Sensor System/Navigation Model/01-Test Model/Navigation Model - Simple/Euler angles & Direction Cosine Using Quaternions/Rotation Angles to DCM1/a22 ==
  normal(q) : Inport
  Demux : Demux
  Product{,1..3} (4 alike) : Product  RndMeth=Zero
  Sum : Sum  Inputs=+-+-
  A22 : Outport
  wires:
  normal(q)/1 -> Demux/1
  Product/1 -> Sum/4
  Product1/1 -> Sum/3
  Product2/1 -> Sum/2
  Product3/1 -> Sum/1
  Demux/1 -> Product3/1, Product3/2
  Demux/2 -> Product2/1, Product2/2
  Demux/3 -> Product1/1, Product1/2
  Demux/4 -> Product/1, Product/2
  Sum/1 -> A22/1

== system AFDNFSmodelSPA/Navigation & Sensor System/Navigation Model/01-Test Model/Navigation Model - Simple/Euler angles & Direction Cosine Using Quaternions/Rotation Angles to DCM1/a23 ==
  normal(q) : Inport
  Demux : Demux
  Gain : Gain  Gain=2
  Product1 : Product  RndMeth=Zero
  Product2 : Product  RndMeth=Zero
  Sum : Sum  Inputs=|++
  A23 : Outport
  wires:
  Demux/4 -> Product2/2
  Product2/1 -> Sum/2
  Product1/1 -> Sum/1
  Sum/1 -> Gain/1
  Demux/1 -> Product1/1
  Demux/2 -> Product1/2
  Demux/3 -> Product2/1
  Gain/1 -> A23/1
  normal(q)/1 -> Demux/1

== system AFDNFSmodelSPA/Navigation & Sensor System/Navigation Model/01-Test Model/Navigation Model - Simple/Euler angles & Direction Cosine Using Quaternions/Rotation Angles to DCM1/a31 ==
  normal(q) : Inport
  Demux : Demux
  Gain : Gain  Gain=2
  Product1 : Product  RndMeth=Zero
  Product2 : Product  RndMeth=Zero
  Sum : Sum  Inputs=|++
  A31 : Outport
  wires:
  Sum/1 -> Gain/1
  Gain/1 -> A31/1
  normal(q)/1 -> Demux/1
  Demux/3 -> Product1/2
  Demux/2 -> Product2/1
  Demux/4 -> Product2/2
  Product2/1 -> Sum/2
  Product1/1 -> Sum/1
  Demux/1 -> Product1/1

== system AFDNFSmodelSPA/Navigation & Sensor System/Navigation Model/01-Test Model/Navigation Model - Simple/Euler angles & Direction Cosine Using Quaternions/Rotation Angles to DCM1/a32 ==
  normal(q) : Inport
  Demux : Demux
  Gain : Gain  Gain=2
  Product1 : Product  RndMeth=Zero
  Product2 : Product  RndMeth=Zero
  Sum : Sum  Inputs=|-+
  A32 : Outport
  wires:
  normal(q)/1 -> Demux/1
  Gain/1 -> A32/1
  Demux/3 -> Product2/1
  Demux/2 -> Product1/2
  Demux/1 -> Product1/1
  Sum/1 -> Gain/1
  Product1/1 -> Sum/1
  Product2/1 -> Sum/2
  Demux/4 -> Product2/2

== system AFDNFSmodelSPA/Navigation & Sensor System/Navigation Model/01-Test Model/Navigation Model - Simple/Euler angles & Direction Cosine Using Quaternions/Rotation Angles to DCM1/a33 ==
  normal(q) : Inport
  Demux : Demux
  Product{,1..3} (4 alike) : Product  RndMeth=Zero
  Sum : Sum  Inputs=+--+
  A33 : Outport
  wires:
  normal(q)/1 -> Demux/1
  Product/1 -> Sum/4
  Product1/1 -> Sum/3
  Product2/1 -> Sum/2
  Product3/1 -> Sum/1
  Demux/1 -> Product3/1, Product3/2
  Demux/2 -> Product2/1, Product2/2
  Demux/3 -> Product1/1, Product1/2
  Demux/4 -> Product/1, Product/2
  Sum/1 -> A33/1

== system AFDNFSmodelSPA/Navigation & Sensor System/Navigation Model/01-Test Model/Navigation Model - Simple/Euler angles & Direction Cosine Using Quaternions/Rotation Angles to Quaternions1/Quaternion Normalize ==
  q : Inport
  Demux : Demux
  Demux1 : Demux
  Mux : Mux
  Product{,1..3} (4 alike) : Product  Inputs=*/
  Product{4..7} (4 alike) : Product
  Sum : Sum  Inputs=4
  sqrt : Sqrt  AlgorithmType=Newton-Raphson  SaturateOnIntegerOverflow=on
  normal(q) : Outport
  wires:
  Product3/1 -> Mux/4
  Product2/1 -> Mux/3
  Product1/1 -> Mux/2
  Product/1 -> Mux/1
  sqrt/1 -> Product3/2, Product2/2, Product/2, Product1/2
  q/1 -> Demux/1, Demux1/1
  Mux/1 -> normal(q)/1
  Demux/1 -> Product/1
  Demux/2 -> Product1/1
  Demux/3 -> Product2/1
  Demux/4 -> Product3/1
  Sum/1 -> sqrt/1
  Product4/1 -> Sum/1
  Product5/1 -> Sum/2
  Product6/1 -> Sum/3
  Product7/1 -> Sum/4
  Demux1/1 -> Product4/2, Product4/1
  Demux1/2 -> Product5/2, Product5/1
  Demux1/3 -> Product6/2, Product6/1
  Demux1/4 -> Product7/2, Product7/1

== system AFDNFSmodelSPA/Nonlinear Flight Simulator/Forces and Moments/Aerodynamic Forces and /Forces/Force Coefficients Calculator/Lift Coefficient/Velocity Magnitude ==
  Velocity : Inport
  Dot Product : DotProduct  InputSameDT=on  OutDataTypeStr=Inherit: Inherit via internal rule
  Sqrt : Sqrt  SaturateOnIntegerOverflow=on
  Velocity Magnitude : Outport
  wires:
  Sqrt/1 -> Velocity Magnitude/1  "abs(V)"
  Velocity/1 -> Dot Product/2, Dot Product/1
  Dot Product/1 -> Sqrt/1

== system AFDNFSmodelSPA/Nonlinear Flight Simulator/Forces and Moments/Aerodynamic Forces and /Forces/Force Coefficients Calculator/SideForce Coefficient/Velocity Magnitude ==
  Velocity : Inport
  Dot Product : DotProduct  InputSameDT=on  OutDataTypeStr=Inherit: Inherit via internal rule
  Sqrt : Sqrt  SaturateOnIntegerOverflow=on
  Velocity Magnitude : Outport
  wires:
  Sqrt/1 -> Velocity Magnitude/1  "abs(V)"
  Velocity/1 -> Dot Product/2, Dot Product/1
  Dot Product/1 -> Sqrt/1

== system AFDNFSmodelSPA/Nonlinear Flight Simulator/Forces and Moments/Aerodynamic Forces and /Turbulence/Turbulence Model/Dryden Turbulence Model/Velocity Magnitude ==
  Velocity : Inport
  Dot Product : DotProduct  InputSameDT=on  OutDataTypeStr=Inherit: Inherit via internal rule
  Sqrt : Sqrt  SaturateOnIntegerOverflow=on
  Velocity Magnitude : Outport
  wires:
  Sqrt/1 -> Velocity Magnitude/1  "abs(V)"
  Velocity/1 -> Dot Product/2, Dot Product/1
  Dot Product/1 -> Sqrt/1

== system AFDNFSmodelSPA/Nonlinear Flight Simulator/Forces and Moments/Aerodynamic Forces and /Turbulence/Turbulence Model/Von-Karman Turbulence Model/Velocity Magnitude ==
  Velocity : Inport
  Dot Product : DotProduct  InputSameDT=on  OutDataTypeStr=Inherit: Inherit via internal rule
  Sqrt : Sqrt  SaturateOnIntegerOverflow=on
  Velocity Magnitude : Outport
  wires:
  Dot Product/1 -> Sqrt/1
  Velocity/1 -> Dot Product/1, Dot Product/2
  Sqrt/1 -> Velocity Magnitude/1  "abs(V)"
